simulink model "Project_Model2020b"  (R2020b)
settings: Solver=FixedStepAuto  StartTime=0.0  StopTime=20  FixedStep=0.001  RelTol=1e-3  AbsTol=1e-3  EnableMultiTasking=on
values from neighbouring files (symbols this model uses):
  constant_mat = [m; mu; r; N]    [Constant_Matrix.m]
  design_mat = design_matrix(ii,:)'    [simRun.m]
libraries: simulink x1
settings Model: Creator=sajal  LastModifiedBy=Srivatsan
settings SolverCC: AutoScaleAbsTol=off
settings DataIOCC: LimitDataPoints=on  MaxDataPoints=10000
settings OptimizationCC: LifeSpan=inf
settings DebuggingCC: AllowSymbolicDim=off  SFUnexpectedBacktrackingDiag=warning  SFNoUnconditionalDefaultTransitionDiag=warning  SFExecutionAtInitializationDiag=none  ArithmeticOperatorsInVariantConditions=warning
settings SFSimCC: SimUseLocalCustomCode=off  CustomCodeUndefinedFunction=UseInterfaceOnly
settings RTWCC: RTWUseLocalCustomCode=off
settings CodeAppCC: StateflowObjectComments=on
settings GRTTargetCC: TargetLangStandard=C89/C90 (ANSI)
settings ConfigComp: CovMetricSettings=dw  CovSaveCumulativeToWorkspaceVar=on  CovSaveSingleToWorkspaceVar=on  CovExternalEMLEnable=off  CovSFcnEnable=off
settings SimscapeCC: SimscapeLogType=all  SimscapeLogSimulationStatistics=on  SimscapeLogDataHistory=10000

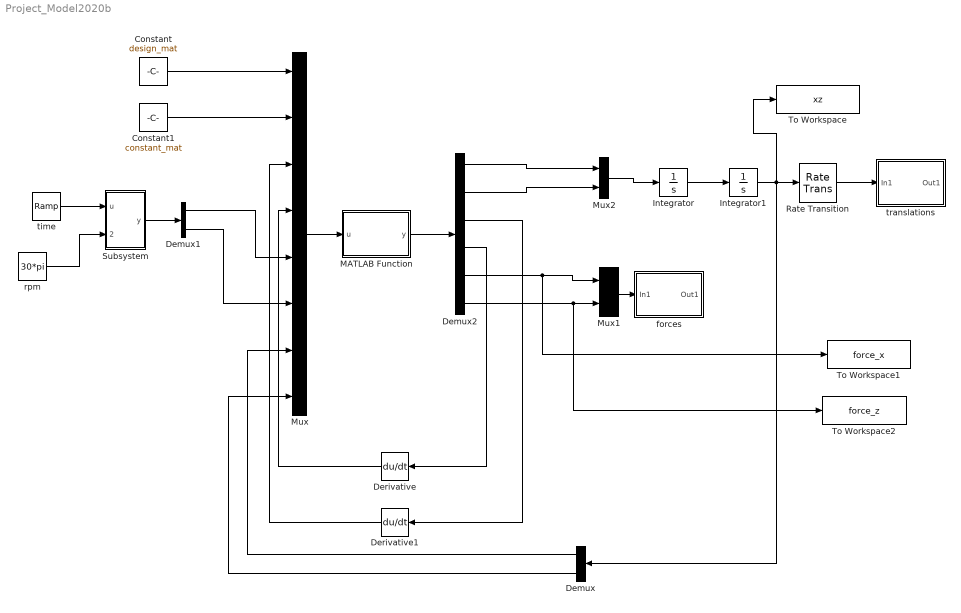
== system Project_Model2020b ==
  Constant : Constant  Value=design_mat
  Constant1 : Constant  Value=constant_mat
  Demux : Demux  Outputs=2
  Demux1 : Demux  Outputs=2
  Demux2 : Demux  Outputs=6
  Derivative : Derivative
  Derivative1 : Derivative
  Integrator : Integrator
  Integrator1 : Integrator
  MATLAB Function : MATLAB Function  TreatAsAtomicUnit=on
  Mux : Mux  Inputs=8
  Mux1 : Mux  Inputs=2
  Mux2 : Mux  Inputs=2
  Rate Transition : RateTransition
  Subsystem : Subsystem
  To Workspace : ToWorkspace  VariableName=xz  SampleTime=-1
  To Workspace1 : ToWorkspace  VariableName=force_x  SampleTime=-1
  To Workspace2 : ToWorkspace  VariableName=force_z  SampleTime=-1
  forces : Subsystem
  rpm : Constant  Value=30*pi
  time : simulink/Sources/Ramp  slope=1  start=0  InitialOutput=0
  translations : Subsystem
  wires:
  time/1 -> Subsystem/1(u)
  Constant/1 -> Mux/1
  Constant1/1 -> Mux/2
  Derivative1/1 -> Mux/3
  Derivative/1 -> Mux/4
  Subsystem/1(y) -> Demux1/1
  Demux1/1 -> Mux/5
  Demux1/2 -> Mux/6
  Mux/1 -> MATLAB Function/1(u)
  MATLAB Function/1(y) -> Demux2/1
  Demux2/5 -> To Workspace1/1, Mux1/1
  Demux2/6 -> To Workspace2/1, Mux1/2
  Demux2/4 -> Derivative/1
  Demux2/3 -> Derivative1/1
  Demux2/1 -> Mux2/1
  Demux2/2 -> Mux2/2
  Mux2/1 -> Integrator/1
  Integrator/1 -> Integrator1/1
  Integrator1/1 -> To Workspace/1, Demux/1, Rate Transition/1
  Demux/1 -> Mux/7
  Demux/2 -> Mux/8
  Mux1/1 -> forces/1(In1)
  Rate Transition/1 -> translations/1(In1)
  rpm/1 -> Subsystem/2(rpm)

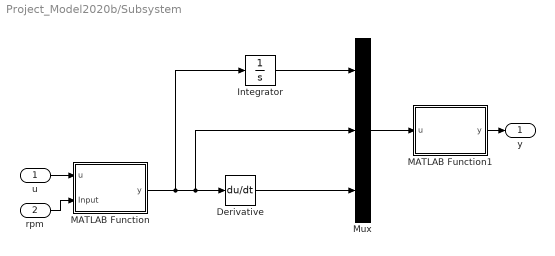
== system Project_Model2020b/Subsystem ==
  u : Inport
  rpm : Inport  Port=2
  Derivative : Derivative
  Integrator : Integrator
  MATLAB Function : MATLAB Function  TreatAsAtomicUnit=on
  MATLAB Function1 : MATLAB Function  TreatAsAtomicUnit=on
  Mux : Mux  Inputs=3
  y : Outport
  wires:
  MATLAB Function1/1(y) -> y/1
  MATLAB Function/1(y) -> Integrator/1, Derivative/1, Mux/2
  Integrator/1 -> Mux/1
  u/1 -> MATLAB Function/1(u)
  Derivative/1 -> Mux/3
  Mux/1 -> MATLAB Function1/1(u)
  rpm/1 -> MATLAB Function/2(Input)

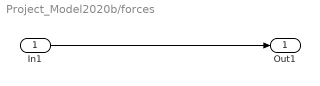
== system Project_Model2020b/forces ==
  In1 : Inport
  Out1 : Outport
  wires:
  In1/1 -> Out1/1

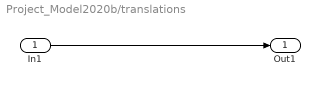
== system Project_Model2020b/translations ==
  In1 : Inport
  Out1 : Outport
  wires:
  In1/1 -> Out1/1

== matlab function Project_Model2020b/Subsystem/MATLAB Function ==
  data: u input; y output; Input input
function y = fcn(u, Input)
y=Input*(1-exp(-u/1.8));  %beta_d'

== matlab function Project_Model2020b/MATLAB Function ==
  data: u input; y output
function y = fcn(u)

y = zeros(6,1);

vd_1 = u(11);
vd_2 = u(12);
Fx_ext = u(13);
Fz_ext = u(14);
x = u(15);
z = u(16);

k = u(1);
c = u(2);
xs1 = u(3);
zs1 = u(4);
xd1 = u(5);
zd1 = u(6);

xs2 = xs1; zs2 = zs1;
xd2 = xd1; zd2 = zd1;

m = u(7);
mu = u(8);
r = u(9);
N = u(10);
% SPRING 1
xs1_d = xs1-x; zs1_d = zs1-z;
ls1 = sqrt(xs1^2+zs1^2);
ls1_d = sqrt(xs1_d^2+zs1_d^2);
Fs1 = (ls1-ls1_d)*k;
Fs1_x = Fs1*xs1_d/ls1_d;
Fs1_z = Fs1*zs1_d/ls1_d;

% SPRING 2
xs2_d = xs2+x; zs2_d = zs2-z;
ls2 = sqrt(xs2^2+zs2^2);
ls2_d = sqrt(xs2_d^2+zs2_d^2);
Fs2 = (ls2-ls2_d)*k;
Fs2_x = Fs2*xs2_d/ls2_d;
Fs2_z = Fs2*zs2_d/ls2_d;

% DAMPER 1
xd1_d = xd1-x; zd1_d = zd1+z;
ld1 = sqrt(xd1^2+zd1^2);
ld1_d = sqrt(xd1_d^2+zd1_d^2);
Fd1 = vd_1*c;
Fd1_x = Fd1*xd1_d/ld1_d;
Fd1_z = Fd1*zd1_d/ld1_d;

% DAMPER 2
xd2_d = xd2+x; zd2_d = zd2+z;
ld2 = sqrt(xd2^2+zd2^2);
ld2_d = sqrt(xd2_d^2+zd2_d^2);
Fd2 = vd_2*c;
Fd2_x = Fd2*xd2_d/ld2_d;
Fd2_z = Fd2*zd2_d/ld2_d;



%FINAL EQUATIONS:
F = [Fx_ext-Fs1_x+Fs2_x+Fd1_x-Fd2_x;...
     Fz_ext-Fs1_z-Fs2_z-Fd1_z-Fd2_z];
 

y(1) = (1/m)*F(1);
y(2) = (1/m)*F(2);

y(3) = ld1_d;
y(4) = ld2_d;

y(5) = F(1);
y(6) = F(2);
end

== matlab function Project_Model2020b/Subsystem/MATLAB Function1 ==
  data: u input; y output
function y = fcn(u)
y=zeros(2,1);
mu = 2; %Unbalanced Mass
r = 0.25; %Radius
beta_d = u(1);
beta_ddot = u(2);
beta_dddot = u(3);
Fn = mu*r*beta_ddot^2;
Ft = mu*r*beta_dddot;
y(1) = Fn*cos(beta_d)-Ft*sin(beta_d);  %Fx_ext
y(2) = Fn*sin(beta_d)+Ft*cos(beta_d);  %Fz_ext
end
